simulink model "faceStringCHL_dev"  (R2018b)
settings: Solver=VariableStepAuto  StartTime=0.0  StopTime=100  RelTol=1e-3
libraries: VCTlbx x1
settings Model: Creator=Ulysses  LastModifiedBy=Ulysses

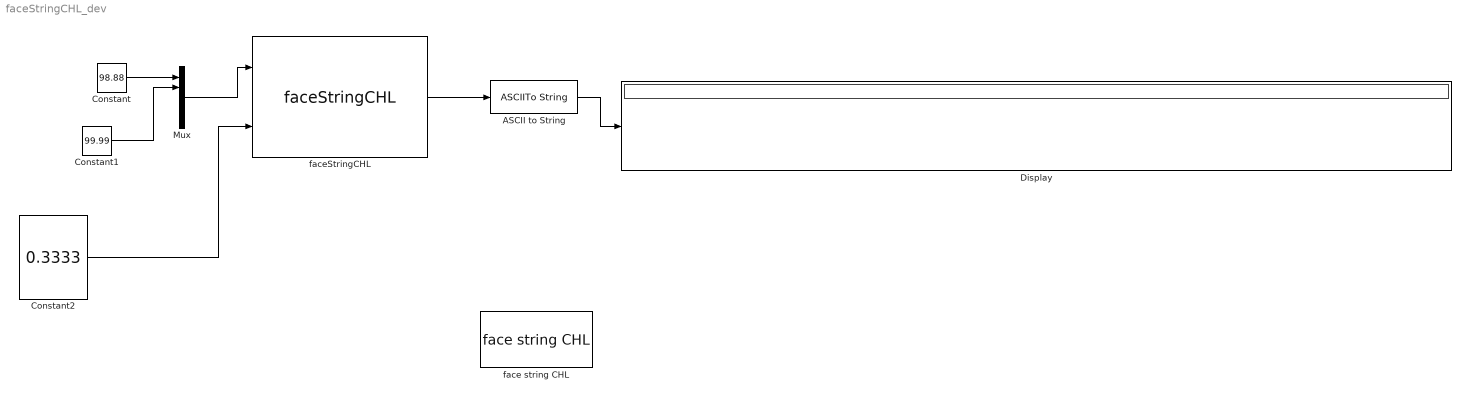
== system faceStringCHL_dev ==
  ASCII to String : ASCIIToString
  Constant : Constant  Value=98.88
  Constant1 : Constant  Value=99.99
  Constant2 : Constant  Value=0.3333
  Display : Display
  Mux : Mux  Inputs=5
  face string CHL : VCTlbx/face string CHL  ActionUnitIDs=[8 9]
      settings: SourceProductName=CHL Toolbox
  faceStringCHL : S-Function  InitFcn=try, set_param(gcb,'FunctionName','faceStringCHL'), end  FunctionName=faceStringCHL  Parameters=uint8(1)  SFunctionModules=faceStringCHL_wrapper faceStringCHL_mycode  SFunctionDeploymentMode=off  EnableBusSupport=off  mask(S-Function Builder){}
      mask help: Simulink:masks:SFunctionBuilder_MD
      mask init:
      | val = [[.9  0.75 0.75 1 1 .9 .9 1]',[1 1 0.75 0.75 .9 .9 1 .9]'];try , sys = get_param(gcb,'SfunBuilderFcnName');if isempty(sys), sys = get_param(gcb,'FunctionName'); end,catch, sys = get_param(gcb,'FunctionName'); end
      settings: CopyFcn=set_param(gcbh,'LinkStatus','none')  PreSaveFcn=try, set_param(gcb,'FunctionName','faceStringCHL'), end  OpenFcn=sfunctionwizard(gcbh)
      mask Display:
      | plot(val(:,1),val(:,2))
      | disp(sys)
      | port_label('input',1,'AUs')
      | port_label('input',2,'duration')
      | port_label('output',1,'faceStrArr')
  wires:
  Mux/1 -> faceStringCHL/1
  Constant/1 -> Mux/1
  faceStringCHL/1 -> ASCII to String/1
  ASCII to String/1 -> Display/1
  Constant1/1 -> Mux/2
  Constant2/1 -> faceStringCHL/2
